simulink model "MPPT"  (R2016a)
settings: Solver=VariableStepAuto  StartTime=0.0  StopTime=5  FixedStep=1e-6  RelTol=1e-3
undefined symbols (not defined in the file or in its folder): sigbuilder_block
libraries: powerlib x19, dsparch4 x4, dspsigops x4, re_lib x2, powerlib_meascontrol x2
settings Model: Creator=Jose  LastModifiedBy=Jose

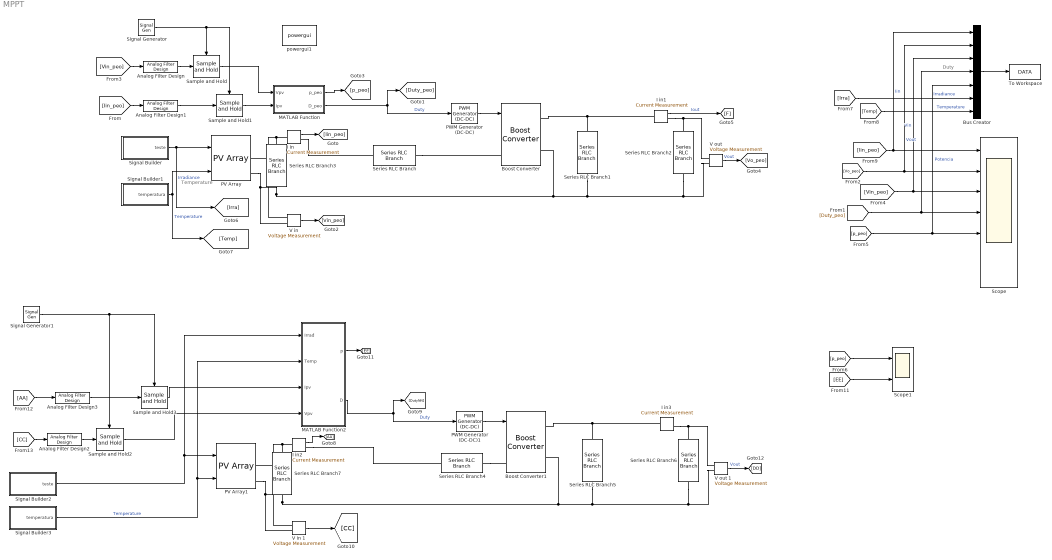
== system MPPT ==
  note: Temperature
  note: Duty
  Analog Filter Design{,1..3} (4 alike) : dsparch4/Analog Filter Design  method=Butterworth  filttype=Lowpass  N=2  Wlo=2*pi*80  Whi=80  Rp=2  Rs=40
  Boost Converter : powerlib/Power Electronics/Boost Converter  ModelType=Switching devices  Ron=0.1  Rs=1e6  Cs=inf  Vforward=[0,0]  Ron_Diode=1e-3  Rs_Diode=1e6  Cs_Diode=inf  Vf_Diode=1e-3  Rs_CurrentSource=inf
  Boost Converter1 : powerlib/Power Electronics/Boost Converter  ModelType=Switching devices  Ron=0.1  Rs=1e6  Cs=inf  Vforward=[0,0]  Ron_Diode=1e-3  Rs_Diode=1e6  Cs_Diode=inf  Vf_Diode=1e-3  Rs_CurrentSource=inf
  Bus Creator : BusCreator  Inputs=7
  I in{,1..3} (4 alike) : powerlib/Measurements/Current Measurement  PhasorSimulation=off  OutputType=Complex  PSBequivalent=0
  MATLAB Function : MATLAB Function  TreatAsAtomicUnit=on
  MATLAB Function2 : MATLAB Function  TreatAsAtomicUnit=on
  PV Array : re_lib/Solar/PV Array  Npar=1  Nser=1  PlotType=array @ 1000 W/m2 & specified temperatures  S_vec="[ 1000  500  100 ]"  Temp_C_vec="[ 45 25  ]"  ModuleName=1Soltech 1STH-215-P  PlotWhenSelected=off  Pm=213.15  Ncell=60  Voc=36.3  Isc=7.84  Vm=29  Im=7.35  beta_Voc_pc=-0.36099  alpha_Isc_pc=0.102  beta_Voc=-0.13104  alpha_Isc=0.007997  IL=7.8649  I0=2.9259e-10  nI=0.98117  Rsh=313.3991  Rs=0.39383  BAL=off  Tc=1e-6  Tfilter=5e-5
  PV Array1 : re_lib/Solar/PV Array  Npar=1  Nser=1  PlotType=array @ 1000 W/m2 & specified temperatures  S_vec="[ 1000  500  100 ]"  Temp_C_vec="[ 45 25  ]"  ModuleName=1Soltech 1STH-215-P  PlotWhenSelected=off  Pm=213.15  Ncell=60  Voc=36.3  Isc=7.84  Vm=29  Im=7.35  beta_Voc_pc=-0.36099  alpha_Isc_pc=0.102  beta_Voc=-0.13104  alpha_Isc=0.007997  IL=7.8649  I0=2.9259e-10  nI=0.98117  Rsh=313.3991  Rs=0.39383  BAL=off  Tc=1e-6  Tfilter=5e-5
  PWM Generator (DC-DC) : powerlib_meascontrol/Pulse & Signal Generators/PWM Generator (DC-DC)  Fsw=20000  Ts=0
  PWM Generator (DC-DC)1 : powerlib_meascontrol/Pulse & Signal Generators/PWM Generator (DC-DC)  Fsw=20000  Ts=0
  Sample and Hold{,1..3} (4 alike) : dspsigops/Sample and Hold  trig=Rising edge  initCond=0  latchinput=off
  Scope : Scope  NumInputPorts=7
  Scope1 : Scope  NumInputPorts=2
  Series RLC Branch : powerlib/Elements/Series RLC Branch  LConnTagsString=__new0  RConnTagsString=__new0  BranchType=L  Resistance=1  Inductance=1300e-6  SetiL0=on  InitialCurrent=7.4  Capacitance=1e-6  Setx0=off  InitialVoltage=0  Measurements=None
  Series RLC Branch1 : powerlib/Elements/Series RLC Branch  LConnTagsString=__new0  RConnTagsString=__new0  BranchType=C  Resistance=1  Inductance=1e-3  SetiL0=off  InitialCurrent=0  Capacitance=680e-6  Setx0=on  InitialVoltage=58  Measurements=None
  Series RLC Branch2 : powerlib/Elements/Series RLC Branch  LConnTagsString=__new0  RConnTagsString=__new0  BranchType=R  Resistance=16  Inductance=1e-3  SetiL0=off  InitialCurrent=0  Capacitance=1e-6  Setx0=off  InitialVoltage=0  Measurements=None
  Series RLC Branch3 : powerlib/Elements/Series RLC Branch  LConnTagsString=__new0  RConnTagsString=__new0  BranchType=C  Resistance=1  Inductance=1e-3  SetiL0=off  InitialCurrent=0  Capacitance=20e-6  Setx0=on  InitialVoltage=29  Measurements=None
  Series RLC Branch4 : powerlib/Elements/Series RLC Branch  LConnTagsString=__new0  RConnTagsString=__new0  BranchType=L  Resistance=1  Inductance=1300e-6  SetiL0=on  InitialCurrent=7.4  Capacitance=1e-6  Setx0=off  InitialVoltage=0  Measurements=None
  Series RLC Branch5 : powerlib/Elements/Series RLC Branch  LConnTagsString=__new0  RConnTagsString=__new0  BranchType=C  Resistance=1  Inductance=1e-3  SetiL0=off  InitialCurrent=0  Capacitance=680e-6  Setx0=on  InitialVoltage=58  Measurements=None
  Series RLC Branch6 : powerlib/Elements/Series RLC Branch  LConnTagsString=__new0  RConnTagsString=__new0  BranchType=R  Resistance=16  Inductance=1e-3  SetiL0=off  InitialCurrent=0  Capacitance=1e-6  Setx0=off  InitialVoltage=0  Measurements=None
  Series RLC Branch7 : powerlib/Elements/Series RLC Branch  LConnTagsString=__new0  RConnTagsString=__new0  BranchType=C  Resistance=1  Inductance=1e-3  SetiL0=off  InitialCurrent=0  Capacitance=20e-6  Setx0=on  InitialVoltage=29  Measurements=None
  Signal Generator : SignalGenerator  WaveForm=square  Frequency=10000
  Signal Generator1 : SignalGenerator  WaveForm=square  Frequency=10000
  Signal Builder : Subsystem  Tag=STV Subsys  LoadFcn=sigbuilder_block('load');  StartFcn=sigbuilder_block('start');  StopFcn=sigbuilder_block('stop');  ClipboardFcn=sigbuilder_block('clipboard');  mask(Sigbuilder block){}
      mask help: Simulink:masks:SigbuilderBlock_MD
      mask init:
      | if ~strcmp(get_param(bdroot(gcbh),'SimulationStatus'),'stopped') tuvar = sigbuilder_block('maskInit'); end
      settings: CopyFcn=sigbuilder_block('copy');  DeleteFcn=sigbuilder_block('delete');  ModelCloseFcn=sigbuilder_block('modelClose');  PreSaveFcn=sigbuilder_block('preSave');  PauseFcn=sigbuilder_block('pause');  ContinueFcn=sigbuilder_block('continue');  NameChangeFcn=sigbuilder_block('namechange');  OpenFcn=sigbuilder_block('open',[153 117 1024.5 489 ]);  CloseFcn=sigbuilder_block('close');
      mask Display: plot(0, 0, 100, 100,[2, 2, 32, 32, 2], [68, 8, 8, 68, 68],[32, 2], [38, 38], [32, 19, 2],[53, 60, 44], [32, 17, 17, 2],[16, 16, 31, 31]);txt = getActiveGroup(gcbh);text(2, 100, txt,'verticalAlignment', 'top');
  Signal Builder1 : Subsystem  Tag=STV Subsys  LoadFcn=sigbuilder_block('load');  StartFcn=sigbuilder_block('start');  StopFcn=sigbuilder_block('stop');  ClipboardFcn=sigbuilder_block('clipboard');  mask(Sigbuilder block){}
      mask help: Simulink:masks:SigbuilderBlock_MD
      mask init:
      | if ~strcmp(get_param(bdroot(gcbh),'SimulationStatus'),'stopped') tuvar = sigbuilder_block('maskInit'); end
      settings: CopyFcn=sigbuilder_block('copy');  DeleteFcn=sigbuilder_block('delete');  ModelCloseFcn=sigbuilder_block('modelClose');  PreSaveFcn=sigbuilder_block('preSave');  PauseFcn=sigbuilder_block('pause');  ContinueFcn=sigbuilder_block('continue');  NameChangeFcn=sigbuilder_block('namechange');  OpenFcn=sigbuilder_block('open',[437.25 153.75 550.5 359.25 ]);  CloseFcn=sigbuilder_block('close');
      mask Display: plot(0, 0, 100, 100,[2, 2, 32, 32, 2], [68, 8, 8, 68, 68],[32, 2], [38, 38], [32, 19, 2],[53, 60, 44], [32, 17, 17, 2],[16, 16, 31, 31]);txt = getActiveGroup(gcbh);text(2, 100, txt,'verticalAlignment', 'top');
  Signal Builder2 : Subsystem  Tag=STV Subsys  LoadFcn=sigbuilder_block('load');  StartFcn=sigbuilder_block('start');  StopFcn=sigbuilder_block('stop');  ClipboardFcn=sigbuilder_block('clipboard');  mask(Sigbuilder block){}
      mask help: Simulink:masks:SigbuilderBlock_MD
      mask init:
      | if ~strcmp(get_param(bdroot(gcbh),'SimulationStatus'),'stopped') tuvar = sigbuilder_block('maskInit'); end
      settings: CopyFcn=sigbuilder_block('copy');  DeleteFcn=sigbuilder_block('delete');  ModelCloseFcn=sigbuilder_block('modelClose');  PreSaveFcn=sigbuilder_block('preSave');  PauseFcn=sigbuilder_block('pause');  ContinueFcn=sigbuilder_block('continue');  NameChangeFcn=sigbuilder_block('namechange');  OpenFcn=sigbuilder_block('open',[6 63.75 1012.5 448.5 ]);  CloseFcn=sigbuilder_block('close');
      mask Display: plot(0, 0, 100, 100,[2, 2, 32, 32, 2], [68, 8, 8, 68, 68],[32, 2], [38, 38], [32, 19, 2],[53, 60, 44], [32, 17, 17, 2],[16, 16, 31, 31]);txt = getActiveGroup(gcbh);text(2, 100, txt,'verticalAlignment', 'top');
  Signal Builder3 : Subsystem  Tag=STV Subsys  LoadFcn=sigbuilder_block('load');  StartFcn=sigbuilder_block('start');  StopFcn=sigbuilder_block('stop');  ClipboardFcn=sigbuilder_block('clipboard');  mask(Sigbuilder block){}
      mask help: Simulink:masks:SigbuilderBlock_MD
      mask init:
      | if ~strcmp(get_param(bdroot(gcbh),'SimulationStatus'),'stopped') tuvar = sigbuilder_block('maskInit'); end
      settings: CopyFcn=sigbuilder_block('copy');  DeleteFcn=sigbuilder_block('delete');  ModelCloseFcn=sigbuilder_block('modelClose');  PreSaveFcn=sigbuilder_block('preSave');  PauseFcn=sigbuilder_block('pause');  ContinueFcn=sigbuilder_block('continue');  NameChangeFcn=sigbuilder_block('namechange');  OpenFcn=sigbuilder_block('open',[437.25 153.75 550.5 359.25 ]);  CloseFcn=sigbuilder_block('close');
      mask Display: plot(0, 0, 100, 100,[2, 2, 32, 32, 2], [68, 8, 8, 68, 68],[32, 2], [38, 38], [32, 19, 2],[53, 60, 44], [32, 17, 17, 2],[16, 16, 31, 31]);txt = getActiveGroup(gcbh);text(2, 100, txt,'verticalAlignment', 'top');
  To Workspace : ToWorkspace  VariableName=DATA  SampleTime=0.25
      settings: Save2DSignal=2-D array (concatenate along first dimension)
  "V in " : powerlib/Measurements/Voltage Measurement  PhasorSimulation=off  OutputType=Complex  PSBequivalent=0
  V in 1 : powerlib/Measurements/Voltage Measurement  PhasorSimulation=off  OutputType=Complex  PSBequivalent=0
  "V out " : powerlib/Measurements/Voltage Measurement  PhasorSimulation=off  OutputType=Complex  PSBequivalent=0
  V out 1 : powerlib/Measurements/Voltage Measurement  PhasorSimulation=off  OutputType=Complex  PSBequivalent=0
  powergui1 : powerlib/powergui  Priority=1  SimulationMode=Continuous  SolverType=Tustin/Backward Euler (TBE)  SampleTime=50e-6  frequency=60  SPID=on  DisableSnubberDevices=off  DisableRonSwitches=on  DisableVfSwitches=on  SwTol=0  DisplayEquations=off  Interpol=off  ExternalGateDelay=off  methode=off  Ts=10  FunctionMessages=off  echomessages=off  HookPort=off  EnableUseOfTLC=off  x0status=blocks  frequencyindice=0  Pbase=100e6  ErrMax=1e-4  Iterations=50  UnitsV=kV  UnitsW=MW  buscounter=0  RestoreLinks=warning  ResistiveCurrentMeasurement=off  Frange=[0:2:500]  Ylog=off  Xlog=on  ShowGrid=off  save=off  variable=ZData  structure=0  ZoomFFT=off  StartTime=0.0  cycles=1  DisplayStyle=1  fundamental=60  FreqAxis=off  MaxFrequency=1000  frequencyindicesteady=1  RmsSteady=1  display=off
  wires:
  PWM Generator (DC-DC)/1 -> Boost Converter/1
  [Iin_peo] -> Bus Creator/1, Scope/1  "Iin"
  I in/1 -> [Iin_peo]
  [Duty_peo] -> Bus Creator/4, Scope/4
  "V in "/1 -> [Vin_peo]
  [Vin_peo] -> Bus Creator/3, Scope/3  "Vin"
  MATLAB Function/1(p_peo) -> [p_peo]
  [p_peo] -> Bus Creator/5, Scope/5  "Potencia"
  "V out "/1 -> [Vo_peo]  "Vout"
  [Vo_peo] -> Bus Creator/2, Scope/2  "Vout"
  MATLAB Function/2(D_peo) -> [Duty_peo], PWM Generator (DC-DC)/1  "Duty"
  I in1/1 -> [F]  "Iout"
  Bus Creator/1 -> To Workspace/1
  Sample and Hold/1 -> MATLAB Function/1(Vpv)
  Sample and Hold1/1 -> MATLAB Function/2(Ipv)
  Signal Generator/1 -> Sample and Hold1/Trigger, Sample and Hold/Trigger
  Analog Filter Design1/1 -> Sample and Hold1/1
  Analog Filter Design/1 -> Sample and Hold/1
  [Vin_peo] -> Analog Filter Design/1
  [Irra] -> Bus Creator/6  "Irradiance"
  [Temp] -> Bus Creator/7  "Temperature"
  Signal Builder1/1(temperatura) -> [Temp], PV Array/2  "Temperature"
  Signal Builder/1(teste) -> PV Array/1, [Irra]  "Irradiance"
  PWM Generator (DC-DC)1/1 -> Boost Converter1/1
  I in2/1 -> [AA]
  V in 1/1 -> [CC]
  MATLAB Function2/1(p) -> [EE]
  V out 1/1 -> [DD]  "Vout"
  MATLAB Function2/2(D) -> PWM Generator (DC-DC)1/1, [DutyNN]  "Duty"
  Sample and Hold2/1 -> MATLAB Function2/4(Vpv)
  Sample and Hold3/1 -> MATLAB Function2/3(Ipv)
  [AA] -> Analog Filter Design3/1
  Signal Generator1/1 -> Sample and Hold3/Trigger, Sample and Hold2/Trigger
  Analog Filter Design3/1 -> Sample and Hold3/1
  Analog Filter Design2/1 -> Sample and Hold2/1
  [CC] -> Analog Filter Design2/1
  Signal Builder3/1(temperatura) -> MATLAB Function2/2(Temp), PV Array1/2  "Temperature"
  Signal Builder2/1(teste) -> MATLAB Function2/1(Irrad), PV Array1/1
  [p_peo] -> Scope1/1
  [EE] -> Scope1/2
  [Iin_peo] -> Analog Filter Design1/1
  connections:
  I in/LConn1 -- "V in "/LConn1 -- PV Array/RConn1 -- Series RLC Branch3/LConn1
  I in1/LConn1 -- Boost Converter/RConn1 -- Series RLC Branch1/LConn1
  Series RLC Branch/RConn1 -- Boost Converter/LConn1
  PV Array/RConn2 -- "V in "/LConn2 -- Series RLC Branch3/RConn1 -- "V out "/LConn2 -- Series RLC Branch2/RConn1 -- Series RLC Branch1/RConn1 -- Boost Converter/RConn2
  I in1/RConn1 -- "V out "/LConn1 -- Series RLC Branch2/LConn1
  I in/RConn1 -- Series RLC Branch/LConn1
  Series RLC Branch7/LConn1 -- I in2/LConn1 -- V in 1/LConn1 -- PV Array1/RConn1
  Series RLC Branch5/LConn1 -- I in3/LConn1 -- Boost Converter1/RConn1
  Boost Converter1/RConn2 -- V out 1/LConn2 -- Series RLC Branch6/RConn1 -- Series RLC Branch5/RConn1 -- Series RLC Branch7/RConn1 -- PV Array1/RConn2 -- V in 1/LConn2
  Series RLC Branch6/LConn1 -- I in3/RConn1 -- V out 1/LConn1
  Series RLC Branch4/RConn1 -- Boost Converter1/LConn1
  I in2/RConn1 -- Series RLC Branch4/LConn1

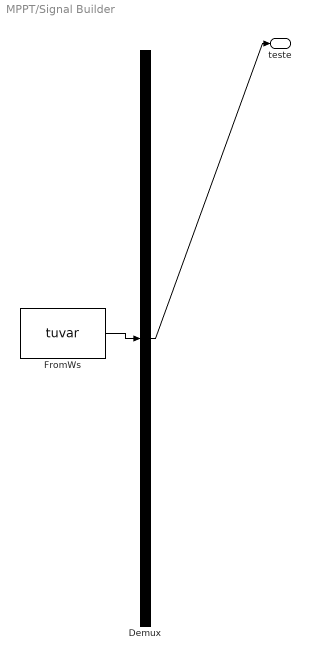
== system MPPT/Signal Builder ==
  Demux : Demux  Tag=STV Demux  Outputs=1
  FromWs : FromWorkspace  Tag=STV FromWs  VariableName=tuvar  SampleTime=0
      SigBuilderData=|
      | common.afterFinalStr = 'Extrapolate'
      | common.sampleTime = 0
      | dataSet.timeRange = [0 3000]
      | dataSet.name = 'Imported_Group 1'
      | sbobj.Name = 'Signal Builder'
      | sbobj.Groups.Name = 'Imported_Group 1'
      | sbobj.Groups.Signals.Name = 'teste'
      | sbobj.Groups.Signals.XData = [0 1 1 2 2 3 3 4 4 5 5 6 ... (5998 elements, 1x5998)]
      | sbobj.Groups.Signals.YData = [1000 1000 836 836 755 755 524 524 905 905 1017 1017 ... (5998 elements, 1x5998)]
      | sbobj.Groups.TimeRange = [0 3000]
  teste : Outport
  wires:
  FromWs/1 -> Demux/1
  Demux/1 -> teste/1

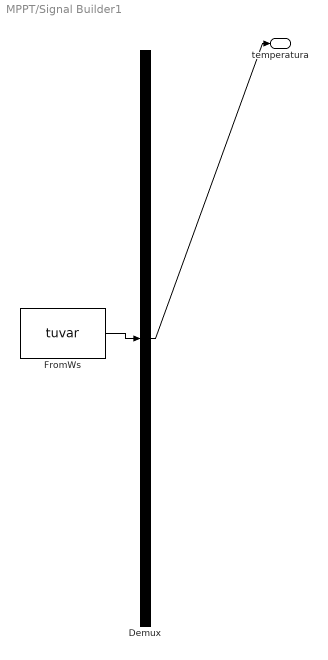
== system MPPT/Signal Builder1 ==
  Demux : Demux  Tag=STV Demux  Outputs=1
  FromWs : FromWorkspace  Tag=STV FromWs  VariableName=tuvar  SampleTime=0
      SigBuilderData=|
      | common.afterFinalStr = 'Extrapolate'
      | common.sampleTime = 0
      | dataSet.timeRange = [0 3000]
      | dataSet.name = 'Imported_Group 1'
      | sbobj.Name = 'Signal Builder'
      | sbobj.Groups.Name = 'Imported_Group 1'
      | sbobj.Groups.Signals.Name = 'temperatura'
      | sbobj.Groups.Signals.XData = [0 0.5 0.5 1.5 1.5 2.5 2.5 3.5 3.5 4.5 4.5 5.5 ... (5945 elements, 1x5945)]
      | sbobj.Groups.Signals.YData = [25 25 60 60 48 48 42 42 55 55 36 36 ... (5945 elements, 1x5945)]
      | sbobj.Groups.TimeRange = [0 3000]
  temperatura : Outport
  wires:
  FromWs/1 -> Demux/1
  Demux/1 -> temperatura/1

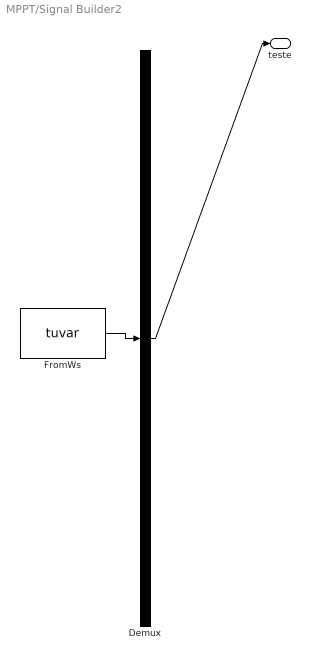
== system MPPT/Signal Builder2 ==
  Demux : Demux  Tag=STV Demux  Outputs=1
  FromWs : FromWorkspace  Tag=STV FromWs  VariableName=tuvar  SampleTime=0
      SigBuilderData=|
      | common.afterFinalStr = 'Extrapolate'
      | common.sampleTime = 0
      | dataSet.timeRange = [0 3000]
      | dataSet.name = 'Imported_Group 1'
      | sbobj.Name = 'Signal Builder'
      | sbobj.Groups.Name = 'Imported_Group 1'
      | sbobj.Groups.Signals.Name = 'teste'
      | sbobj.Groups.Signals.XData = [0 1 1 2 2 3 3 4 4 5 5 6 ... (5998 elements, 1x5998)]
      | sbobj.Groups.Signals.YData = [1000 1000 836 836 755 755 524 524 905 905 1017 1017 ... (5998 elements, 1x5998)]
      | sbobj.Groups.TimeRange = [0 3000]
  teste : Outport
  wires:
  FromWs/1 -> Demux/1
  Demux/1 -> teste/1

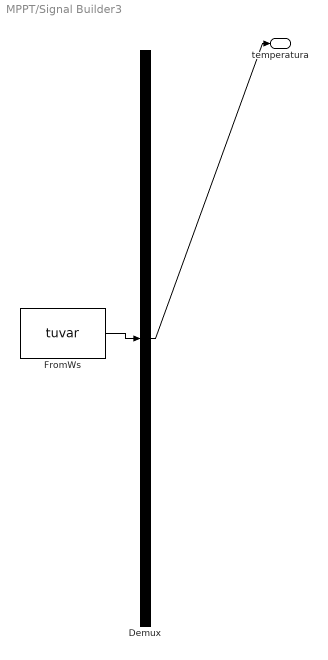
== system MPPT/Signal Builder3 ==
  Demux : Demux  Tag=STV Demux  Outputs=1
  FromWs : FromWorkspace  Tag=STV FromWs  VariableName=tuvar  SampleTime=0
      SigBuilderData=|
      | common.afterFinalStr = 'Extrapolate'
      | common.sampleTime = 0
      | dataSet.timeRange = [0 3000]
      | dataSet.name = 'Imported_Group 1'
      | sbobj.Name = 'Signal Builder'
      | sbobj.Groups.Name = 'Imported_Group 1'
      | sbobj.Groups.Signals.Name = 'temperatura'
      | sbobj.Groups.Signals.XData = [0 0.5 0.5 1.5 1.5 2.5 2.5 3.5 3.5 4.5 4.5 5.5 ... (5945 elements, 1x5945)]
      | sbobj.Groups.Signals.YData = [25 25 60 60 48 48 42 42 55 55 36 36 ... (5945 elements, 1x5945)]
      | sbobj.Groups.TimeRange = [0 3000]
  temperatura : Outport
  wires:
  FromWs/1 -> Demux/1
  Demux/1 -> temperatura/1

== matlab function MPPT/MATLAB Function ==
  data: p_peo output; Vpv input; D_peo output; Ipv input
function [p_peo,D_peo] = PandO(Vpv,Ipv)
%#codegen
% ************************************************************
% MATLAB implementation of a Perturb and Observe algorithm
% for Maximum Power Point Tracking. This algorithm is designed
% to operate with a buck converter
%
% Created by: José
% ************************************************************

% Define internal values for the voltage and power as persistent
% variables
persistent Dprev Pprev Vprev

% Initialize the internal values for the voltage and power on the
% first pass
if isempty(Dprev)
    Dprev = 0.5;
    Vprev = 30;
    Pprev = 200;
end

% Initialize algorithm parameters
deltaD = 0.001;

% Calculate measured array power
Ppv = Vpv*Ipv;
p_peo=Ppv;
% Increase or decrease duty cycle based on conditions
if (Ppv-Pprev) ~= 0
    if (Ppv-Pprev) > 0
        if (Vpv-Vprev) > 0
            D_peo = Dprev - deltaD;
        else
            D_peo = Dprev + deltaD;
        end
    else
        if (Vpv-Vprev) > 0
            D_peo = Dprev + deltaD;
        else
            D_peo = Dprev - deltaD;
        end        
    end
else
    
    D_peo = Dprev;
    
end

% Update internal values
Dprev = D_peo;
Vprev = Vpv;
Pprev = Ppv;

== matlab function MPPT/MATLAB Function2 ==
  data: Irrad input; p output; Temp input; Ipv input; Vpv input; D output
function [p, D] = NeuralNetwork( Irrad, Temp, Ipv, Vpv)

persistent pesos bias mean_ std_ x_norm X1 X2 Neu Neu2
pesos = [0.251217909485928 -0.478535784614218 0.548078848564446 0.120260246679279 0.186582709037477 0.402969057923924 -0.231948239872258 -0.257714780265481 -0.732324592715146;0.953903246235852 -0.352008204316699 -0.133946462125217 -0.0184680852487036 0.294782267055285 0.442235623378212 0.815081468008676 -0.380286167396861 -0.105464652676165;0.625653400141098 0.0674994575566867 -0.0502531351525982 -0.275460359490919 -0.725051291084327 0.227141698128815 0.123650725746100 -0.119647401461989 -0.0130381976802497;0.550676212911902 -0.0835844638098857 -0.151075367132844 0.0537258312746533 0.179844590632326 -0.418134255730516 0.848505261431117 0.786748602366608 -0.361787295695965];
bias = [-0.239808857111034;-0.322634196818954;0.879646423811435;-0.137265964642077;-0.689791001260579;0.461624809368098;0.134800775467773;-0.203619664796477;-0.245028187406052];

if isempty(Dprev)
    x_norm = [0.005860859503435 -0.050248966113807 0.713760914431750 0.444185058536029];
    X1 = [0 0 0 0];
    Neu = 0;
    X2 = [0 0 0 0];
    Neu2 = 0;
end

x = [ Irrad  Temp  Ipv  Vpv ];
W1= pesos(:,1:4);
W2= pesos(:,5:8);
WO= pesos(:,9);
b1= bias(1:4,:);
b2= bias(5:8,:);
b3= bias(9,:);
p = Ipv*Vpv;

mean_=[730.65487572  35.59751434   5.14613337  27.86261631];
std_=[4.59565912e+04 2.10900147e+02 2.34331624e+00 4.32227478e+00];

for i=1:4
    x_norm(i) =(x(i) - mean_(i))/std_(i);
end

for i=1:4
    Neu =  dot( x_norm ,W1(1:4,i)) ; %Produto interno
    X1(1,i)  = tanh( Neu + b1(i,1))   ;
end
for i=1:1:4 % 5 to 8
    Neu2 =  dot( X1 , ( W2(1:4,i) ) ) ;
    X2(1,i)  =  tanh( Neu2 + b2(i,1) )  ;
end

D = ( dot( X2,(WO) ) + b3 );
